simulink model "pdcontrol_org"  (Simulink 10.0)
settings: Solver=ode45  StartTime=0.0  StopTime=5  RelTol=1e-3  EnableMultiTasking=on
InitFcn:
  | param
undefined symbols (not defined in the file): AP
settings Model: Creator=paul  LastModifiedBy=bhisma
settings DataIOCC: LimitDataPoints=on
settings DebuggingCC: SolverPrmCheckMsg=warning
settings GRTTargetCC: GeneratePreprocessorConditionals=Disable all  CombineOutputUpdateFcns=on  GRTInterface=off
settings ConfigComp: CovExternalEMLEnable=off

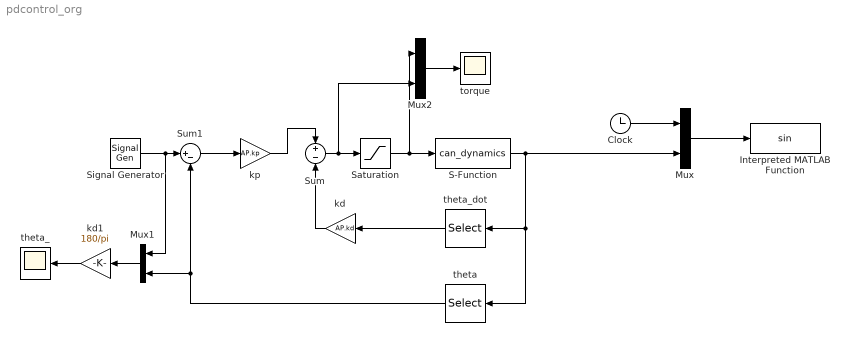
== system pdcontrol_org ==
  Clock : Clock
  Interpreted MATLAB Function : MATLABFcn  OutputDimensions=0  SampleTime=0.01
  Mux : Mux  Inputs=2
  Mux1 : Mux  Inputs=2
  Mux2 : Mux  Inputs=2
  S-Function : S-Function  FunctionName=can_dynamics  Parameters=AP  SFunctionDeploymentMode=off  EnableBusSupport=off
  Saturation : Saturate  UpperLimit=AP.F_max  LowerLimit=-AP.F_max  SampleTime=AP.Ts
  Signal Generator : SignalGenerator  Amplitude=pi/3
  Sum : Sum  Inputs=+-
  Sum1 : Sum  Inputs=|+-  SampleTime=AP.Ts
  kd : Gain  Gain=AP.kd
  kd1 : Gain  Gain=180/pi
  kp : Gain  Gain=AP.kp
  theta : Selector  InputPortWidth=2  IndexOptions=Index vector (dialog)  Indices=1  OutputSizes=1
  theta_ : Scope
  theta_dot : Selector  InputPortWidth=2  IndexOptions=Index vector (dialog)  Indices=2  OutputSizes=1
  torque : Scope
  wires:
  Signal Generator/1 -> Mux1/1, Sum1/1
  Sum1/1 -> kp/1
  kp/1 -> Sum/1
  Clock/1 -> Mux/1
  S-Function/1 -> theta_dot/1, theta/1, Mux/2
  Mux/1 -> Interpreted MATLAB Function/1
  kd/1 -> Sum/2
  theta_dot/1 -> kd/1
  theta/1 -> Mux1/2, Sum1/2
  kd1/1 -> theta_/1
  Mux1/1 -> kd1/1
  Sum/1 -> Saturation/1, Mux2/2
  Mux2/1 -> torque/1
  Saturation/1 -> Mux2/1, S-Function/1
